simulink model "es601_ex01"  (R2019a)
settings: Solver=VariableStepAuto  StartTime=0.0  StopTime=11.0  RelTol=1e-3
settings Model: Creator=Admin-PC  LastModifiedBy=Admin-PC

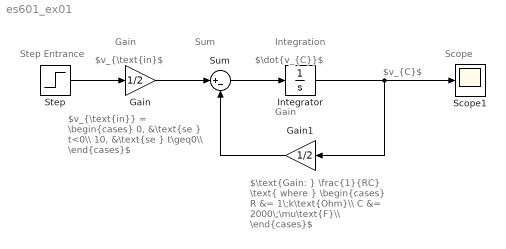
== system es601_ex01 ==
  note: $v_{C}$
  note: $\dot{v_{C}}$
  note: $v_{\text{in}$
  note: $v_{\text{in}} = \begin{cases} 0, &\text{se } t<0\\ 10, &\text{se } t\geq0\\ \end{cases}$
  note: $\text{Gain: } \frac{1}{RC} \text{ where } \begin{cases} R &= 1\;k\text{Ohm}\\ C &= 2000\;\mu\text{F}\\ \end{cases}$
  note: Step Entrance
  note: Integration
  note: Gain
  note: Gain
  note: Sum
  note: Scope
  Gain : Gain  Gain=1/2
  Gain1 : Gain  Gain=1/2
  Integrator : Integrator
  Scope1 : Scope
  Step : Step  Time=0  After=10  SampleTime=0
  Sum : Sum  Inputs=|+-
  wires:
  Step/1 -> Gain/1
  Integrator/1 -> Scope1/1, Gain1/1
  Gain/1 -> Sum/1
  Sum/1 -> Integrator/1
  Gain1/1 -> Sum/2
